simulink library "Pump_basic"  (Simulink 8.2)
settings: Solver=ode45  StartTime=0.0  StopTime=10.0  RelTol=1e-3
undefined symbols (not defined in the file): ID, MassFlow, Temperature
libraries: carnot x1
settings Model: Creator=lena.frank  LastModifiedBy=drhf

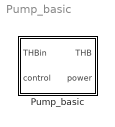
== system Pump_basic ==
  Pump_basic : Subsystem  mask(basic Pump){mdotmax=1200/3600, fluid_id=1, mix=0, dia=0.02, power=30, p0=3e5, hgt=0, ID=ID}
      mask prompts: mdotmax "massflow rate [kg/s]"; fluid_id "fluid"; mix "percentage of fluid mix [0..1]"; dia "diameter at in- and outlet [m]"; power "electric power consumption [W]"; p0 "system pressure [Pa]"; hgt "static height in m (positive value above ground)"; ID "ID (pressure drop calculation mode)"
      mask help:
      | Set constant massflow rate according to the control signal.
      | The pump is a very basic model, sometimes creating algebraic loops. If you have problems with algebraic loops, use "Pump_const" instead.
      | ID for pressure drop calculation:
      |     1    .. 9999 No Pressure Drop
      |     10001..19999 Pressure Drop from Massflow
      |     20001..inf   Full Pressure Drop with Static Height
      mask init:
      | mix = min(1, max(0, mix));
      | dia = max(0.001, dia);
      mask Help: web(fullfile(path_carnot('help'),'Pump_basic.html'),'-helpbrowser')
      mask Display: plot(0,0,100,100,[40,70,40,30,30,40,60,70,70,60,40],[70,50,30,40,60,70,70,60,40,30,30])

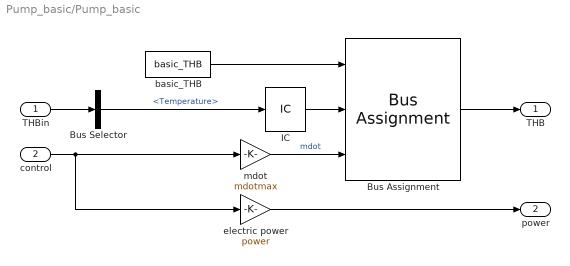
== system Pump_basic/Pump_basic ==
  THBin : Inport
  control : Inport  Port=2
  Bus Assignment : BusAssignment  AssignedSignals=Temperature,MassFlow
  Bus Selector : BusSelector  OutputSignals=Temperature
  IC : InitialCondition  Value=20
  basic_THB : carnot/Basic/Hydraulics/basic_THB  t=20  mdot=0  p=p0  ID=ID  fluid=fluid_id  mix=mix  dia=dia  hgt=hgt
  electric power : Gain  Gain=power  SaturateOnIntegerOverflow=on  OutDataTypeStr=Inherit: Same as input  ParamDataTypeStr=Inherit: Same as input
  mdot : Gain  Gain=mdotmax  SaturateOnIntegerOverflow=on  OutDataTypeStr=Inherit: Same as input  ParamDataTypeStr=Inherit: Same as input
  THB : Outport
  power : Outport  Port=2
  wires:
  IC/1 -> Bus Assignment/2
  mdot/1 -> Bus Assignment/3  "mdot"
  control/1 -> mdot/1, electric power/1
  electric power/1 -> power/1
  THBin/1 -> Bus Selector/1
  Bus Selector/1 -> IC/1  "<Temperature>"
  basic_THB/1 -> Bus Assignment/1
  Bus Assignment/1 -> THB/1
